simulink model "filter_sim_surge_test"  (R2024b)
settings: Solver=VariableStepAuto  StartTime=0.0  StopTime=0.00006  RelTol=1e-3  AbsTol=1e-3
libraries: fl_lib x8, nesl_utility x5, ee_lib x4
settings Model: Creator=micha_l7o089j  LastModifiedBy=micha
settings SolverCC: AutoScaleAbsTol=off  MaxConsecutiveMinStep=10  AlgebraicLoopSolver=TrustRegion  MaxZcPerStep=1
settings DebuggingCC: UnconnectedInputMsg=warning  UnconnectedOutputMsg=warning  UnconnectedLineMsg=warning  SymbolicDimsDataTypeCodeGenerationDiagnostic=none
settings ModelReferenceCC: EnableRefExpFcnMdlSchedulingChecks=on
settings SFSimCC: CustomCodeUndefinedFunction=UseInterfaceOnly
settings RTWCC: GPUComputeCapability=3.5  DLArmComputeVersion=19.05
settings SimscapeCC: SimscapeLogType=all  SimscapeLogSimulationStatistics=on  SimscapeLogDataHistory=10000

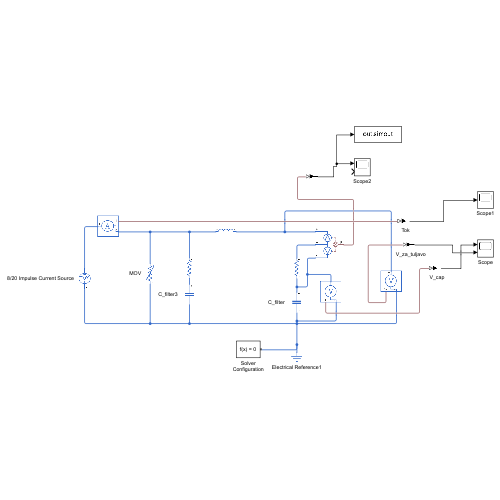
[thumbnail: Simulink's stored preview of the top-level diagram]
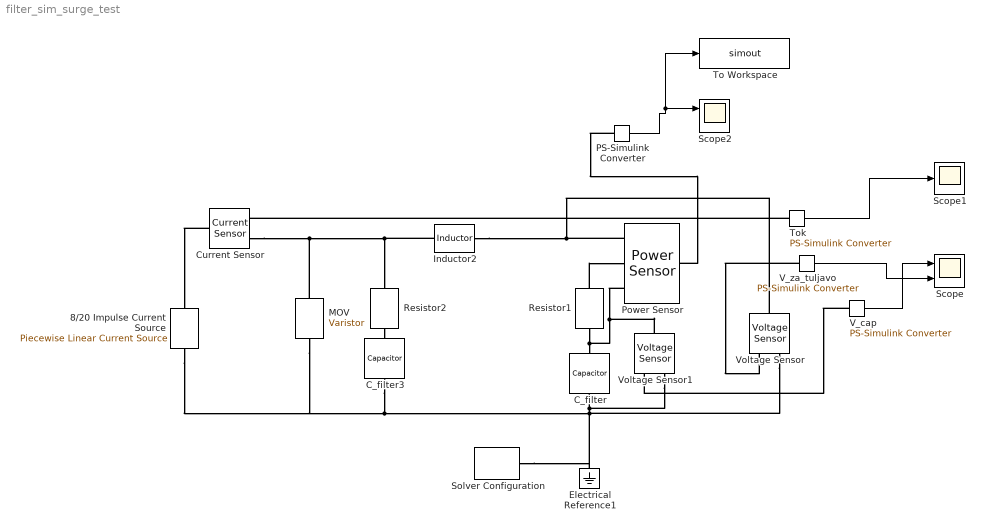
== system filter_sim_surge_test ==
  " 8/20 Impulse Current Source" : ee_lib/Additional Components/SPICE Sources/Piecewise Linear Current Source  TIMElist=|  CURRlist=|  INTERP=2  EXTRAP=2  Gmin_param=ee.enum.gminParam.no
      TIMElist=|
      | [0.0, 0.6060606060606061, 1.2121212121212122, 1.8181818181818183, 2.4242424242424243, 3.0303030303030303, 3.6363636363636367, 4.242424242424242, 4.848484848484849, 5.454545454545455, 6.0606060606060606, 6.666666666666667, 7.272727272727273, 7.878787878787879, 8.484848484848484, 9.090909090909092, 9.696969696969697, 10.303030303030303, 10.90909090909091, 11.515151515151516, 12.121212121212121, 12.727272727272728, 13.333333333333334, 13.93939393939394, 14.545454545454547, 15.151515151515152, 15.757575757575758, 16.363636363636363, 16.96969696969697, 17.575757575757578, 18.181818181818183, 18.78787878787879, 19.393939393939394, 20.0, 20.606060606060606, 21.21212121212121, 21.81818181818182, 22.424242424242426, 23.03030303030303, 23.636363636363637, 24.242424242424242, 24.848484848484848, 25.454545454545457, 26.060606060606062, 26.666666666666668, 27.272727272727273, 27.87878787878788, 28.484848484848484, 29.090909090909093, 29.6969696969697, 30.303030303030305, 30.90909090909091, 31.515151515151516, 32.121212121212125, 32.72727272727273, 33.333333333333336, 33.93939393939394, 34.54545454545455, 35.151515151515156, 35.75757575757576, 36.36363636363637, 36.96969696969697, 37.57575757575758, 38.18181818181818, 38.78787878787879, 39.3939393939394, 40.0, 40.60606060606061, 41.21212121212121, 41.81818181818182, 42.42424242424242, 43.03030303030303, 43.63636363636364, 44.24242424242424, 44.84848484848485, 45.45454545454545, 46.06060606060606, 46.66666666666667, 47.27272727272727, 47.87878787878788, 48.484848484848484, 49.09090909090909, 49.696969696969695, 50.303030303030305, 50.909090909090914, 51.515151515151516, 52.121212121212125, 52.72727272727273, 53.333333333333336, 53.93939393939394, 54.54545454545455, 55.151515151515156, 55.75757575757576, 56.36363636363637, 56.96969696969697, 57.57575757575758, 58.18181818181819, 58.78787878787879, 59.3939393939394, 60.0]
      |  us
      CURRlist=|
      | [0.0, 11620.689207613834, 22579.27148983156, 32847.647015505856, 42403.06743376326, 51227.990134162406, 59309.910497601704, 66641.1742175186, 73218.77177710761, 79044.11716233623, 84122.81287311485, 88464.40326676685, 92082.11822965782, 94992.60912521751, 97215.6789103695, 98774.00824833229, 99692.87937463784, 99999.89939579203, 99724.72461704059, 98898.78740795724, 97555.02702277918, 95727.6256973089, 93451.7512464874, 90763.3072871087, 87698.69210925674, 84294.56711853127, 80587.63566960525, 76614.43301069012, 72411.1279586265, 68013.33682607138, 63455.950026093866, 58772.97168585799, 53997.37251036335, 49160.956049795204, 44294.238440233516, 39426.341607572176, 34584.89984875999, 29795.979633106654, 25084.012399582323, 20471.740063922938, 15980.172892043844, 11628.559343842366, 7434.367443980527, 3413.277193697072, -420.8164999074722, -4055.790933379181, -7481.273339360884, -10688.609849273598, -13670.826312033174, -16422.58160862545, -18940.11411203951, -21221.18194755794, -23264.997709912288, -25072.15829152264, -26644.57047016401, -27985.37289515519, -29098.85509877164, -29990.374144278216, -30666.269503991294, -31133.776740357884, -31400.940540417334, -31476.527629433956, -31369.940063193935, -31091.129370684936, -30650.51198985474, -30058.886409105442, -29327.352396343147, -28467.232665986303, -27489.9973025466, -26407.1912274326, -25230.364963680517, -23971.008921565037, -22640.4913966605, -21250.000441062857, -19810.489738297998, -18332.628583065736, -16826.756038526706, -15302.839316446109, -13770.436399262084, -12238.66289814092, -10716.163117391165, -9211.08527330242, -7731.060794607335, -6283.187612380384, -4874.017329320279, -3509.5461420346082, -2195.2093751722086, -935.8794730327163, 264.1327173813293, 1401.0735480280625, 2471.739240971971, 3473.4658208960614, 4404.1165065324685, 5262.066762819869, 6046.187218491532, 6755.824655385473, 7390.781276104927, 7951.292455807504, 8438.003181928676, 8851.943382619493]
      |  A
      settings: LibrarySourceBlock=ee_lib/Sources/Piecewise Linear Current Source  InternalSimscapePortConfiguration="{\"Bottom\":[],\"Left\":[{\"id\":\"p\",\"label\":\"+\",\"type\":\"foundation.electrical.electrical\"}],\"Right\":[{\"id\":\"n\",\"label\":\"-\",\"type\":\"foundation.electrical.electrical\"}],\"Top\":[]}"
  C_filter : fl_lib/Electrical/Electrical Elements/Capacitor  c=4.7e-6 F  r=1e-6 Ohm  g=0 1/Ohm  i_specify=on  i_priority=None  i=0 A  i_nominal_specify=off  i_nominal_value=1  i_nominal_unit=A  v_specify=on  v_priority=None  v=0 V  v_nominal_specify=off  v_nominal_value=1  v_nominal_unit=V  vc_specify=on  vc_priority=High  vc=0 V  vc_nominal_specify=off  vc_nominal_value=1  vc_nominal_unit=V
  C_filter3 : fl_lib/Electrical/Electrical Elements/Capacitor  c=4.7e-6 F  r=1e-6 Ohm  g=0 1/Ohm  i_specify=on  i_priority=None  i=0 A  i_nominal_specify=off  i_nominal_value=1  i_nominal_unit=A  v_specify=on  v_priority=None  v=0 V  v_nominal_specify=off  v_nominal_value=1  v_nominal_unit=V  vc_specify=on  vc_priority=High  vc=0 V  vc_nominal_specify=off  vc_nominal_value=1  vc_nominal_unit=V
  Current Sensor : fl_lib/Electrical/Electrical Sensors/Current Sensor
  Electrical Reference1 : fl_lib/Electrical/Electrical Elements/Electrical Reference
  Inductor2 : ee_lib/Passive/Inductor  l=100e-6 H  enable_L_tol=ee.enum.toleranceApplication.none  L_tol=20  tol_distribution=ee.enum.toleranceDistribution.uniform  nSigma=4  r=0 Ohm  g=1e-9 1/Ohm  enable_operating_limits=ee.enum.enable.no  operating_limit_action=ee.enum.passive.reportOpLim.warn  max_working_current=1 A  power_rating=1 W  fault_action=simscape.enum.assert.action.none  t_fault=1 s  i_L_specify=off  i_L_priority=High  i_L=0 A  i_L_nominal_specify=off  i_L_nominal_value=1  i_L_nominal_unit=A
  MOV : ee_lib/Passive/Varistor  prm=ee.enum.passive.varistor.varistorParameterization.linear  vclamp=2000 V  roff=10e8 Ohm  ron=2 mOhm  vln=130 V  vnu=300 V  rLeak=3e8 Ohm  alphaNormal=45  rUpturn=0.07 Ohm  rseries=100e-6 Ohm  c=4.4 nF  v_varistor_specify=on  v_varistor_priority=None  v_varistor=0 V  v_varistor_nominal_specify=on  v_varistor_nominal_value=1  v_varistor_nominal_unit=V
      settings: InternalSimscapePortConfiguration="{\"Bottom\":[],\"Left\":[{\"id\":\"p\",\"label\":\"+\",\"type\":\"foundation.electrical.electrical\"}],\"Right\":[{\"id\":\"n\",\"label\":\"-\",\"type\":\"foundation.electrical.electrical\"}],\"Top\":[]}"
  PS-Simulink Converter : nesl_utility/PS-Simulink Converter  PhysicalDomain=network_engine_domain  SubClassName=ps_output  LeftPortType=input  RightPortType=output  PseudoPeriodic=off  Frequencies=[]  VectorFormat=inherit  Unit=inherit  AffineConversion=off
  Power Sensor : ee_lib/Sensors & Transducers/Power Sensor  measurement_type=1  averaging_period=1e-4 s
  Resistor1 : fl_lib/Electrical/Electrical Elements/Resistor  R=1 mOhm  i_specify=off  i_priority=None  i=0 A  i_nominal_specify=off  i_nominal_value=1  i_nominal_unit=A  v_specify=off  v_priority=None  v=0 V  v_nominal_specify=off  v_nominal_value=1  v_nominal_unit=V
  Resistor2 : fl_lib/Electrical/Electrical Elements/Resistor  R=10 Ohm  i_specify=off  i_priority=None  i=0 A  i_nominal_specify=off  i_nominal_value=1  i_nominal_unit=A  v_specify=off  v_priority=None  v=0 V  v_nominal_specify=off  v_nominal_value=1  v_nominal_unit=V
  Scope : Scope  NumInputPorts=2
  Scope1 : Scope
  Scope2 : Scope  NumInputPorts=2
  Solver Configuration : nesl_utility/Solver Configuration  PhysicalDomain=network_engine_domain  SubClassName=solver  LeftPortType=input  RightPortType=generic  Tones=[]  Harmonics=[]  SimulateNoise=off  Profile=off  UseLocalSampling=off  EnableSwitchedLinearOptims=on  FrequencyDomain=off  UseCCode=off  RelTol=0.001  AbsTol=1e-06  MinStep=1e-09  ToWorkspace=off  RevertToSquareIcSolve=off  NumHomotopyIterations=100  PhasorMode=off  PhasorModeNumHarmonics=1  ConsistencySolver=NEWTON_XTOL_AFTER_FTOL  IndexReductionMethod=DerivativeReplacement  DoDC=on  ResidualTolerance=1e-09  ConsistencyTolSource=GLOBAL  ConsistencyAbsTol=0.001  ConsistencyRelTol=0.001  ConsistencyTolFactor=0.00001  UseLocalSolver=off  LocalSolverChoice=NE_BACKWARD_EULER_ADVANCER  ResolveIndetEquations=on  FunctionEvalNumThread=1  LocalSolverSampleTime=0.000001  DoFixedCost=off  MaxNonlinIter=3  MaxModeIter=2  ComputeImpulses=off  ImpulseIterations=2  LinearAlgebra=Full  LinearAlgebraNumThread=0  EquationFormulation=NE_TIME_EF  DelaysMemoryBudget=1024  AutomaticFiltering=on  FilteringTimeConstant=0.001  PartitionStorageMethod=AS_NEEDED  PartitionMemoryBudget=1024  PartitionMethod=ROBUST  MultibodyUseLocalSolver=on  MultibodyLocalSolverChoice=ODE1  MultibodyLocalSolverSampleTime=0.001
  To Workspace : ToWorkspace  VariableName=simout  SaveFormat=Timeseries  SampleTime=-1
  Tok : nesl_utility/PS-Simulink Converter  PhysicalDomain=network_engine_domain  SubClassName=ps_output  LeftPortType=input  RightPortType=output  PseudoPeriodic=off  Frequencies=[]  VectorFormat=inherit  Unit=inherit  AffineConversion=off
  V_cap : nesl_utility/PS-Simulink Converter  PhysicalDomain=network_engine_domain  SubClassName=ps_output  LeftPortType=input  RightPortType=output  PseudoPeriodic=off  Frequencies=[]  VectorFormat=inherit  Unit=inherit  AffineConversion=off
  V_za_tuljavo : nesl_utility/PS-Simulink Converter  PhysicalDomain=network_engine_domain  SubClassName=ps_output  LeftPortType=input  RightPortType=output  PseudoPeriodic=off  Frequencies=[]  VectorFormat=inherit  Unit=inherit  AffineConversion=off
  Voltage Sensor : fl_lib/Electrical/Electrical Sensors/Voltage Sensor
  Voltage Sensor1 : fl_lib/Electrical/Electrical Sensors/Voltage Sensor
  wires:
  V_za_tuljavo/1 -> Scope/2
  V_cap/1 -> Scope/1
  Tok/1 -> Scope1/1
  PS-Simulink Converter/1 -> To Workspace/1, Scope2/1
  connections:
  C_filter3/RConn1 -- " 8/20 Impulse Current Source"/LConn1 -- MOV/RConn1 -- Electrical Reference1/LConn1 -- Solver Configuration/RConn1 -- Voltage Sensor/RConn2 -- C_filter/RConn1 -- Voltage Sensor1/RConn2
  Power Sensor/LConn3 -- C_filter/LConn1 -- Resistor1/RConn1 -- Voltage Sensor1/LConn1
  Power Sensor/LConn1 -- Inductor2/RConn1 -- Voltage Sensor/LConn1
  V_za_tuljavo/LConn1 -- Voltage Sensor/RConn1
  V_cap/LConn1 -- Voltage Sensor1/RConn1
  Tok/LConn1 -- Current Sensor/RConn1
  Resistor1/LConn1 -- Power Sensor/LConn2
  PS-Simulink Converter/LConn1 -- Power Sensor/RConn1
  Resistor2/RConn1 -- C_filter3/LConn1
  Current Sensor/RConn2 -- MOV/LConn1 -- Inductor2/LConn1 -- Resistor2/LConn1
  Current Sensor/LConn1 -- " 8/20 Impulse Current Source"/RConn1
